simulink model "lqr_first"  (R2023b)
settings: Solver=VariableStepAuto  StartTime=0.0  StopTime=20  FixedStep=0.1  RelTol=1e-3
values from neighbouring files (symbols this model uses):
  K = lqr(A,B,Q,R)    [LQR_first.m]
settings Model: Creator=Asus  LastModifiedBy=Asus

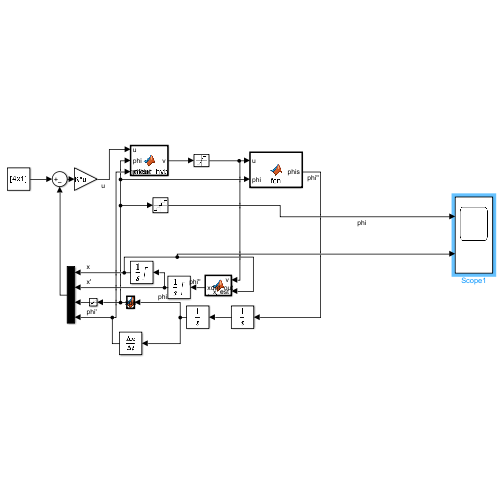
[thumbnail: Simulink's stored preview of the top-level diagram]
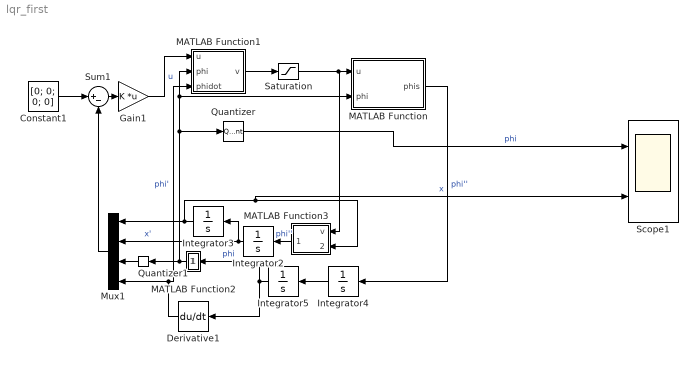
== system lqr_first ==
  Constant1 : Constant  Value=[0; 0; 0; 0]
  Derivative1 : Derivative
  Gain1 : Gain  Gain=K  Multiplication=Matrix(K*u)
  Integrator2 : Integrator  LimitOutput=on  UpperSaturationLimit=2  LowerSaturationLimit=-2
  Integrator3 : Integrator  LimitOutput=on  UpperSaturationLimit=0.4  LowerSaturationLimit=-0.4
  Integrator4 : Integrator
  Integrator5 : Integrator  InitialCondition=3.14
  MATLAB Function : MATLAB Function  TreatAsAtomicUnit=on
  MATLAB Function1 : MATLAB Function  TreatAsAtomicUnit=on
  MATLAB Function2 : MATLAB Function  TreatAsAtomicUnit=on
  MATLAB Function3 : MATLAB Function  TreatAsAtomicUnit=on
  Mux1 : Mux
  Quantizer : Quantizer  QuantizationInterval=2*pi/1600
  Quantizer1 : Quantizer  QuantizationInterval=2*pi/1600
  Saturation : Saturate  UpperLimit=5  LowerLimit=-5
  Scope1 : Scope  NumInputPorts=2
  Sum1 : Sum  Inputs=|+-
  wires:
  Sum1/1 -> Gain1/1
  Constant1/1 -> Sum1/1
  Mux1/1 -> Sum1/2
  Derivative1/1 -> Mux1/4, MATLAB Function1/3(phidot)  "phi'"
  Integrator2/1 -> Integrator3/1, Mux1/2  "x'"
  Integrator3/1 -> MATLAB Function3/2(x_est), Scope1/2, Mux1/1  "x"
  MATLAB Function/1(phis) -> Integrator4/1  "phi''"
  Integrator4/1 -> Integrator5/1
  Integrator5/1 -> MATLAB Function2/1(phi), Derivative1/1  "phi"
  Gain1/1 -> MATLAB Function1/1(u)  "u"
  MATLAB Function1/1(v) -> Saturation/1
  Saturation/1 -> MATLAB Function3/1(v), MATLAB Function/1(u)
  Quantizer/1 -> Scope1/1  "phi"
  MATLAB Function2/1(phi_eq) -> Quantizer1/1, MATLAB Function/2(phi), MATLAB Function1/2(phi), Quantizer/1
  Quantizer1/1 -> Mux1/3
  MATLAB Function3/1(xdot_out) -> Integrator2/1  "phi''"

== matlab function lqr_first/MATLAB Function1 ==
  data: u input; phi input; v output; phidot input
function v = controleur_hybride(u,phi,phidot)
  phi_eq = atan2(sin(phi), cos(phi));   % ramène phi dans [-pi, pi], équivalent physique
    if abs(phi_eq) < pi/3  && abs(phidot) < 2
        v =u;
    else
        g = 9.81; L = 0.5; m = 0.03; 
        E = 0.5*m*L^2*phidot^2 + m*g*L*(cos(phi));
        E_des = m*g*L;  % énergie nécessaire pour atteindre le sommet
        k_swing = 12; % gain à régler expérimentalement
        v = -k_swing * sign(phidot*cos(phi)) * (E_des - E);
    end
end

== matlab function lqr_first/MATLAB Function ==
  data: u input; phis output; phi input
function phis = fcn(u,phi)
    g = 9.81;
    L = 0.5;
    phis= (g*sin(phi) - u*cos(phi)) / L;
end

== matlab function lqr_first/MATLAB Function2 ==
  data: phi input; phi_eq output
function phi_eq= conversion(phi)
  phi_eq = atan2(sin(phi), cos(phi));   % ramène phi dans [-pi, pi], équivalent physique
end

== matlab function lqr_first/MATLAB Function3 ==
  data: v input; xdot_out output; x_est input
function xdot_out = anti_windup_check(v, x_est)
    if (x_est >= 0.38 && v >=0) || (x_est <= -0.38 && v <= 0)
        xdot_out = 0;   % on bloque l'intégration dans le sens qui aggrave
    else
        xdot_out = v;   % sinon, comportement normal
    end
end
